simulink model "is95fwdchdetection2"  (Simulink 4.00)
settings: Solver=VariableStepDiscrete  SolverMode=SingleTasking  StartTime=0.0  StopTime=2  RelTol=1e-3  AbsTol=1e-6
undefined symbols (not defined in the file or in its folder): slcm
libraries: cdmaprivate x8, cdmalibv1p1 x6, commutil2 x4, dspsigattribs x2, commchan2 x2, dspbuff3 x1, commsink2 x1
settings Model: CovMetricSettings=d  Creator=rkumar  LastModifiedBy=akansal  SaveTime=off  SaveOutput=off  LimitDataPoints=off  ExtModeTrigMode=oneshot  ExtModeArmWhenConnect=off  BlockReductionOpt=off

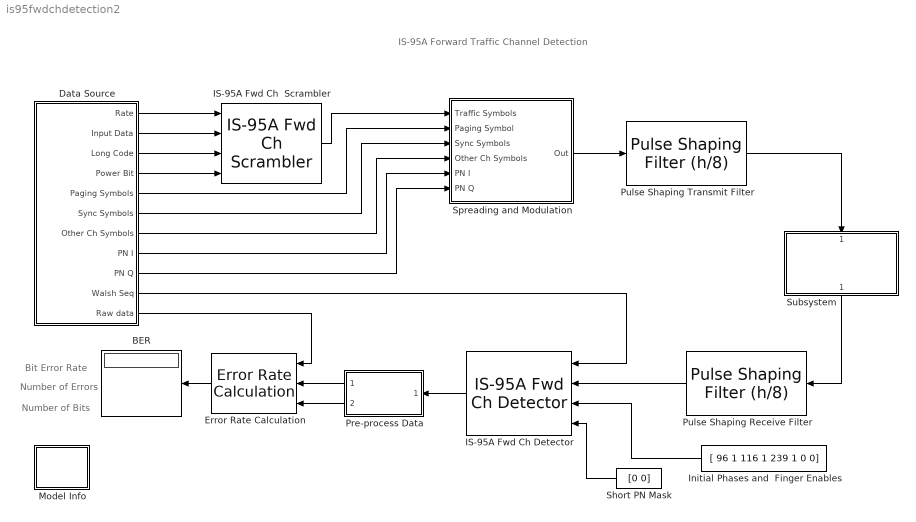
== system is95fwdchdetection2 ==
  note: IS-95A Forward Traffic Channel Detection
  note: Bit Error Rate
  note: Number of Errors
  note: Number of Bits
  BER : Display
      settings: Format=short
  Data Source : Subsystem
      settings: RTWFcnNameOpts=Auto  RTWFileNameOpts=Auto
  Error Rate Calculation : commsink2/Error Rate Calculation  Orientation=left  N=2*384  st_delay=2*384  cp_mode=Select samples from port  subframe=[]  PMode=Port  WsName=ErrorVec  RsMode2=off
  IS-95A Fwd Ch  Scrambler : cdmalibv1p1/IS-95A Base Station Transmitter/IS-95A Fwd Ch Scrambler  rate_set=Rate Set I  chType=Traffic
  IS-95A Fwd Ch Detector : cdmalibv1p1/IS-95A Mobile Station Receiver/IS-95A Fwd Ch Detector  Orientation=left  rateSet=Rate Set I  numSymb=1  wlshOrd=6  rake_buff_size=3  rake_oversamp=8  sampTime=1/(50*384)
  Initial Phases and  Finger Enables : Constant  Orientation=left  Value=[ 96 1 116 1 239 1 0 0]
  Model Info : Subsystem  LoadFcn=slcm LoadBlock;  InitFcn=slcm('UpdateAllCMBlocksInThisModelInit')  mask(CMBlock){InitialSaveTempField=, InitialBlockCM=none, BlockCM=none, Frame=on, SaveTempField=, DisplayStringWithTags=Info, MaskDisplayString=Info, HorizontalTextAlignment=Center, LeftAlignmentValue=0.5, SourceBlockDiagram=is95fwdchdetection2, TagMaxNumber=20, CMTag1=, CMTag2=, CMTag3=, CMTag4=, CMTag5=, CMTag6=, CMTag7=, CMTag8=, CMTag9=, CMTag10=, CMTag11=, CMTag12=, CMTag13=, CMTag14=, CMTag15=, CMTag16=, CMTag17=, CMTag18=, CMTag19=, CMTag20=}
      mask help: This block allows revision control information to be displayed within the model.
      settings: CopyFcn=slcm CopyBlock;  DeleteFcn=slcm Cancel;  PostSaveFcn=slcm('UpdateAllCMBlocksInThisModel')  NameChangeFcn=slcm Rename;  OpenFcn=cdmademohelp;  RTWFcnNameOpts=Auto  RTWFileNameOpts=Auto
      mask Display: text(str2num(LeftAlignmentValue), 0.5, MaskDisplayString, 'HorizontalAlignment', HorizontalTextAlignment)
  Pre-process Data : Subsystem  Orientation=left
      settings: RTWFcnNameOpts=Auto  RTWFileNameOpts=Auto
  Pulse Shaping Receive Filter : cdmaprivate/Pulse Shaping Filter (h//8)  Orientation=left  N=1
  Pulse Shaping Transmit Filter : cdmaprivate/Pulse Shaping Filter (h//8)  N=8
  Short PN Mask : Constant  Orientation=left  Value=[0 0]
  Spreading and Modulation : Subsystem
      settings: RTWFcnNameOpts=Auto  RTWFileNameOpts=Auto
  Subsystem : Subsystem  Orientation=down
      settings: RTWFcnNameOpts=Auto  RTWFileNameOpts=Auto
      mask Display: disp('Rayleigh Multipath\n and  AWGN\nChannel')
  wires:
  Data Source/4(Power Bit) -> IS-95A Fwd Ch  Scrambler/4
  Data Source/1(Rate) -> IS-95A Fwd Ch  Scrambler/1
  Data Source/3(Long Code) -> IS-95A Fwd Ch  Scrambler/3
  Data Source/8(PN I) -> Spreading and Modulation/5(PN I)
  Data Source/9(PN Q) -> Spreading and Modulation/6(PN Q)
  Data Source/7(Other Ch Symbols) -> Spreading and Modulation/4(Other Ch Symbols)
  Data Source/2(Input Data) -> IS-95A Fwd Ch  Scrambler/2
  IS-95A Fwd Ch  Scrambler/1 -> Spreading and Modulation/1(Traffic Symbols)
  Data Source/5(Paging Symbols) -> Spreading and Modulation/2(Paging Symbol)
  Data Source/6(Sync Symbols) -> Spreading and Modulation/3(Sync Symbols)
  Pre-process Data/2(Data Idx) -> Error Rate Calculation/3
  Pre-process Data/1(Hard Data) -> Error Rate Calculation/2
  Error Rate Calculation/1 -> BER/1
  Data Source/11(Raw data) -> Error Rate Calculation/1
  Spreading and Modulation/1("Out ") -> Pulse Shaping Transmit Filter/1
  Pulse Shaping Transmit Filter/1 -> Subsystem/1(" ")
  Short PN Mask/1 -> IS-95A Fwd Ch Detector/4
  IS-95A Fwd Ch Detector/1 -> Pre-process Data/1(Soft Data)
  Data Source/10(Walsh Seq) -> IS-95A Fwd Ch Detector/1
  Pulse Shaping Receive Filter/1 -> IS-95A Fwd Ch Detector/2
  Initial Phases and  Finger Enables/1 -> IS-95A Fwd Ch Detector/3
  Subsystem/1("  ") -> Pulse Shaping Receive Filter/1

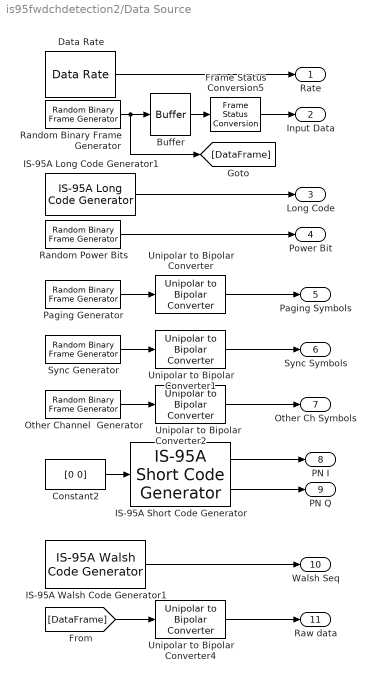
== system is95fwdchdetection2/Data Source ==
  Buffer : dspbuff3/Buffer  N=1  V=0  ic=0
  Constant2 : Constant  Value=[0 0]
  Data Rate : cdmaprivate/Data Rate  rate=Full
  Frame Status Conversion5 : dspsigattribs/Frame Status Conversion  growRefPort=off  outframe=Frame-based
  IS-95A Long Code Generator1 : cdmalibv1p1/IS-95A Common/IS-95A Long Code Generator  num_symb=1  tx_lc_dec_ratio=64  tx_lc_init_mask=2^41  tx_lc_init_state=2^41  tx_sample_time=1/(50*384)
  IS-95A Short Code Generator : cdmalibv1p1/IS-95A Common/IS-95A Short Code Generator  numOut=64  sampTime=1/(50*384)
  IS-95A Walsh Code Generator1 : cdmalibv1p1/IS-95A Common/IS-95A Walsh Code Generator  wlshOrd=6  wlshIndices=38  st=1/(50*384)
  Other Channel  Generator : cdmaprivate/Random Binary Frame Generator  seed=98767657  Ts=1/(50*384)  N=1
  Paging Generator : cdmaprivate/Random Binary Frame Generator  seed=76767  Ts=1/(50*384)  N=1
  Random Binary Frame Generator : cdmaprivate/Random Binary Frame Generator  seed=8514519  Ts=1/(50*384)  N=384
  Random Power Bits : cdmaprivate/Random Binary Frame Generator  seed=8514519  Ts=1/(50*16)  N=1
  Sync Generator : cdmaprivate/Random Binary Frame Generator  seed=465789  Ts=4 * 1/(50*384)  N=1
  Unipolar to Bipolar Converter{,1..2,4} (4 alike) : commutil2/Unipolar to Bipolar Converter  M=2  polarity=Negative
  Rate : Outport  Port=1  InitialOutput=0
  Input Data : Outport  Port=2  InitialOutput=0
  Long Code : Outport  Port=3  InitialOutput=0
  Power Bit : Outport  Port=4  InitialOutput=0
  Paging Symbols : Outport  Port=5  InitialOutput=0
  Sync Symbols : Outport  Port=6  InitialOutput=0
  Other Ch Symbols : Outport  Port=7  InitialOutput=0
  PN I : Outport  Port=8  InitialOutput=0
  PN Q : Outport  Port=9  InitialOutput=0
  Walsh Seq : Outport  Port=10  InitialOutput=0
  Raw data : Outport  Port=11  InitialOutput=0
  wires:
  Data Rate/1 -> Rate/1
  Random Binary Frame Generator/1 -> [DataFrame], Buffer/1
  Random Power Bits/1 -> Power Bit/1
  Constant2/1 -> IS-95A Short Code Generator/1
  Sync Generator/1 -> Unipolar to Bipolar Converter1/1
  Other Channel  Generator/1 -> Unipolar to Bipolar Converter2/1
  Paging Generator/1 -> Unipolar to Bipolar Converter/1
  Unipolar to Bipolar Converter/1 -> Paging Symbols/1
  Unipolar to Bipolar Converter1/1 -> Sync Symbols/1
  Unipolar to Bipolar Converter2/1 -> Other Ch Symbols/1
  Unipolar to Bipolar Converter4/1 -> Raw data/1
  [DataFrame] -> Unipolar to Bipolar Converter4/1
  IS-95A Walsh Code Generator1/1 -> Walsh Seq/1
  Buffer/1 -> Frame Status Conversion5/1
  Frame Status Conversion5/1 -> Input Data/1
  IS-95A Long Code Generator1/1 -> Long Code/1
  IS-95A Short Code Generator/1 -> PN I/1
  IS-95A Short Code Generator/2 -> PN Q/1

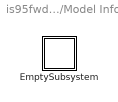
== system is95fwdchdetection2/Model Info ==
  EmptySubsystem : Subsystem
      settings: RTWFcnNameOpts=Auto  RTWFileNameOpts=Auto

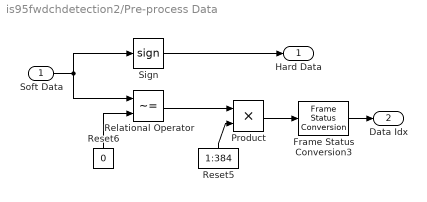
== system is95fwdchdetection2/Pre-process Data ==
  Soft Data : Inport  Port=1
  Frame Status Conversion3 : dspsigattribs/Frame Status Conversion  growRefPort=off  outframe=Sample-based
  Product : Product  Inputs=2  Multiplication=Element-wise(.*)  SaturateOnIntegerOverflow=on
  Relational Operator : RelationalOperator  Operator=~=
  Reset5 : Constant  Orientation=up  Value=1:384
  Reset6 : Constant  Orientation=up  Value=0
  Sign : Signum
  Hard Data : Outport  Port=1
  Data Idx : Outport  Port=2
  wires:
  Product/1 -> Frame Status Conversion3/1
  Reset5/1 -> Product/2
  Relational Operator/1 -> Product/1
  Soft Data/1 -> Sign/1, Relational Operator/1
  Sign/1 -> Hard Data/1
  Reset6/1 -> Relational Operator/2
  Frame Status Conversion3/1 -> Data Idx/1

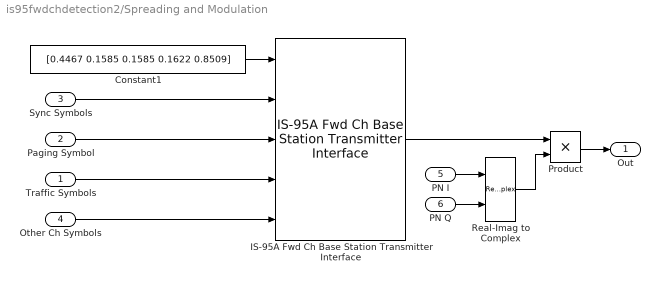
== system is95fwdchdetection2/Spreading and Modulation ==
  Traffic Symbols : Inport  Port=1
  Paging Symbol : Inport  Port=2
  Sync Symbols : Inport  Port=3
  Other Ch Symbols : Inport  Port=4
  PN I : Inport  Port=5
  PN Q : Inport  Port=6
  Constant1 : Constant  Value=[0.4467 0.1585 0.1585 0.1622 0.8509]
  IS-95A Fwd Ch Base Station Transmitter Interface : cdmalibv1p1/IS-95A Base Station Transmitter/IS-95A Fwd Ch Base Station Transmitter Interface  paging_rate=Full  wlshOrd=6  wlsh_indices=[0 32 47 38 23]  sampTime=1/(50*384)
  Product : Product  Inputs=2  Multiplication=Element-wise(.*)  SaturateOnIntegerOverflow=on
  Real-Imag to Complex : RealImagToComplex  Input=RealAndImag  ConstantPart=0
  "Out " : Outport  Port=1  InitialOutput=0
  wires:
  Paging Symbol/1 -> IS-95A Fwd Ch Base Station Transmitter Interface/3
  Traffic Symbols/1 -> IS-95A Fwd Ch Base Station Transmitter Interface/4
  Other Ch Symbols/1 -> IS-95A Fwd Ch Base Station Transmitter Interface/5
  Constant1/1 -> IS-95A Fwd Ch Base Station Transmitter Interface/1
  Sync Symbols/1 -> IS-95A Fwd Ch Base Station Transmitter Interface/2
  PN Q/1 -> Real-Imag to Complex/2
  PN I/1 -> Real-Imag to Complex/1
  Real-Imag to Complex/1 -> Product/2
  IS-95A Fwd Ch Base Station Transmitter Interface/1 -> Product/1
  Product/1 -> "Out "/1

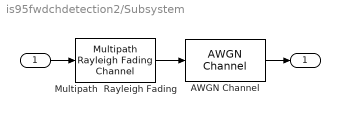
== system is95fwdchdetection2/Subsystem ==
  " " : Inport  Port=1
  AWGN Channel : commchan2/AWGN Channel  seed=123456  noiseMode="Signal to noise ratio  (Es/No)"  EsNodB=12  SNRdB=10  Ps=2  Tsym=1/1228800  variance=1
  "Multipath  Rayleigh Fading " : commchan2/Multipath Rayleigh Fading Channel  Fd=175.92  simTs=1/(1228800*8)  delayVec=[0 2e-6 14.5e-6]  gainVecdB=[0 0 -3]  normGain=on  Seed=83102
  "  " : Outport  Port=1
  wires:
  AWGN Channel/1 -> "  "/1
  " "/1 -> "Multipath  Rayleigh Fading "/1
  "Multipath  Rayleigh Fading "/1 -> AWGN Channel/1

== system is95fwdchdetection2/Model Info/EmptySubsystem ==
